simulink model "IEEE_1547_UI_TEST"  (R2018b)
settings: Solver=ode4  StartTime=0.0  StopTime=inf  FixedStep=Ts  RelTol=1e-3  EnableMultiTasking=on
PostLoadFcn:
  | Ts=40e-6; ARTEMIS_DISABLE_RTLAB_COMPATIBILTY_CHECK=1;
InitFcn:
  | Ts=40e-6; ARTEMIS_DISABLE_RTLAB_COMPATIBILTY_CHECK=1;
undefined symbols (not defined in the file or in its folder): another_event_name, I, Left, my_event_name, Right, type, V
libraries: simulink x72, powerlib_meascontrol x70, powerlib x66, artemis x4, rtlab x3, rtio_opalrt_ml605ex1 x3
(part 3 of 3)

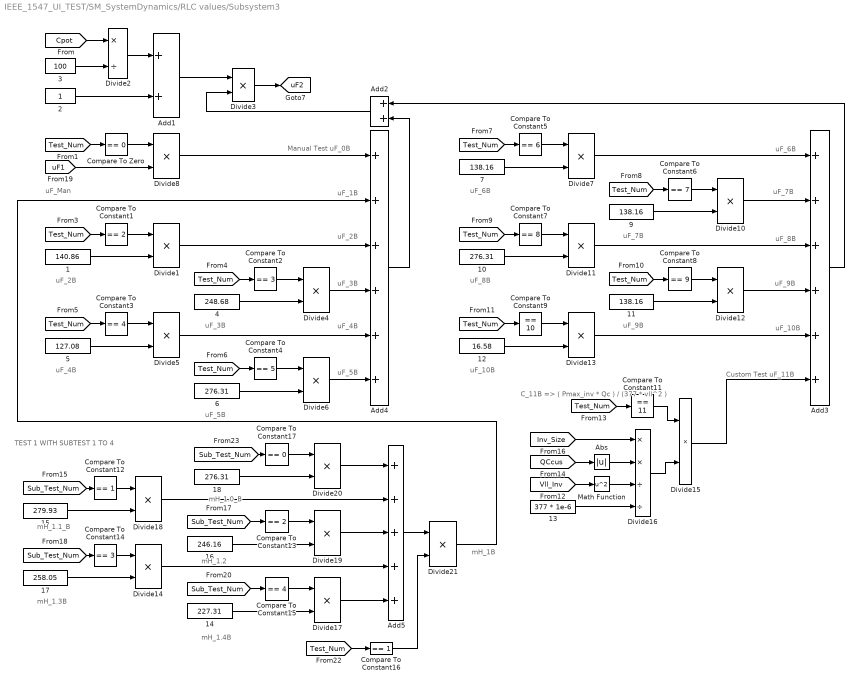
== system IEEE_1547_UI_TEST/SM_SystemDynamics/RLC values/Subsystem3 ==
  note: uF_8B
  note: uF_7B
  note: Manual Test uF_0B
  note: Custom Test uF_11B
  note: uF_2B
  note: uF_7B
  note: mH_1B
  note: uF_8B
  note: uF_5B
  note: C_11B => ( Pmax_inv * Qc ) / (377 * vll^2 )
  note: uF_6B
  note: uF_Man
  note: mH_1.0_B
  note: uF_4B
  note: uF_10B
  note: mH_1.3B
  note: uF_4B
  note: uF_9B
  note: mH_1.2
  note: mH_1.4B
  note: uF_2B
  note: TEST 1 WITH SUBTEST 1 TO 4
  note: uF_9B
  note: uF_5B
  note: uF_10B
  note: uF_6B
  note: uF_3B
  note: uF_3B
  note: mH_1.1_B
  note: uF_1B
  1 : Constant  Value=140.86
  10 : Constant  Value=276.31
  11 : Constant  Value=138.16
  12 : Constant  Value=16.58
  13 : Constant  Value=377 * 1e-6
  14 : Constant  Value=227.31
  15 : Constant  Value=279.93
  16 : Constant  Value=246.16
  17 : Constant  Value=258.05
  18 : Constant  Value=276.31
  2 : Constant
  3 : Constant  Value=100
  4 : Constant  Value=248.68
  5 : Constant  Value=127.08
  6 : Constant  Value=276.31
  7 : Constant  Value=138.16
  9 : Constant  Value=138.16
  Abs : Abs
  Add1 : Sum
  Add2 : Sum
  Add3 : Sum  Inputs=++++++
  Add4 : Sum  Inputs=++++++
  Add5 : Sum  Inputs=+++++
  Compare To Constant1 : simulink/Logic and Bit Operations/Compare To Constant  relop===  const=2  OutDataTypeStr=boolean
  Compare To Constant11 : simulink/Logic and Bit Operations/Compare To Constant  relop===  const=11  OutDataTypeStr=boolean
  Compare To Constant12 : simulink/Logic and Bit Operations/Compare To Constant  relop===  const=1  OutDataTypeStr=boolean
  Compare To Constant13 : simulink/Logic and Bit Operations/Compare To Constant  relop===  const=2  OutDataTypeStr=boolean
  Compare To Constant14 : simulink/Logic and Bit Operations/Compare To Constant  relop===  const=3  OutDataTypeStr=boolean
  Compare To Constant15 : simulink/Logic and Bit Operations/Compare To Constant  relop===  const=4  OutDataTypeStr=boolean
  Compare To Constant16 : simulink/Logic and Bit Operations/Compare To Constant  relop===  const=1  OutDataTypeStr=boolean
  Compare To Constant17 : simulink/Logic and Bit Operations/Compare To Constant  relop===  const=0  OutDataTypeStr=boolean
  Compare To Constant2 : simulink/Logic and Bit Operations/Compare To Constant  relop===  const=3  OutDataTypeStr=boolean
  Compare To Constant3 : simulink/Logic and Bit Operations/Compare To Constant  relop===  const=4  OutDataTypeStr=boolean
  Compare To Constant4 : simulink/Logic and Bit Operations/Compare To Constant  relop===  const=5  OutDataTypeStr=boolean
  Compare To Constant5 : simulink/Logic and Bit Operations/Compare To Constant  relop===  const=6  OutDataTypeStr=boolean
  Compare To Constant6 : simulink/Logic and Bit Operations/Compare To Constant  relop===  const=7  OutDataTypeStr=boolean
  Compare To Constant7 : simulink/Logic and Bit Operations/Compare To Constant  relop===  const=8  OutDataTypeStr=boolean
  Compare To Constant8 : simulink/Logic and Bit Operations/Compare To Constant  relop===  const=9  OutDataTypeStr=boolean
  Compare To Constant9 : simulink/Logic and Bit Operations/Compare To Constant  relop===  const=10  OutDataTypeStr=boolean
  Compare To Zero : simulink/Logic and Bit Operations/Compare To Zero  relop===  OutDataTypeStr=boolean
  Divide{1,3..8,10..15,17..21} (18 alike) : Product  Inputs=**
  Divide16 : Product  Inputs=**//
  Divide2 : Product  Inputs=*/
  Math Function : Math  Operator=square  SaturateOnIntegerOverflow=on
  tag scope: uF2=global
  wires:
  [Test_Num] -> Compare To Constant9/1
  Compare To Constant5/1 -> Divide7/1
  Divide3/1 -> [uF2]
  [Sub_Test_Num] -> Compare To Constant15/1
  Divide21/1 -> Add4/2
  Divide17/1 -> Add5/5
  [Test_Num] -> Compare To Constant7/1
  Divide19/1 -> Add5/3
  11/1 -> Divide12/2
  Compare To Constant17/1 -> Divide20/1
  14/1 -> Divide17/2
  Compare To Constant16/1 -> Divide21/2
  Add5/1 -> Divide21/1
  5/1 -> Divide5/2
  Divide12/1 -> Add3/4
  Divide8/1 -> Add4/1
  Compare To Constant14/1 -> Divide14/1
  Compare To Constant6/1 -> Divide10/1
  16/1 -> Divide19/2
  15/1 -> Divide18/2
  Compare To Constant12/1 -> Divide18/1
  13/1 -> Divide16/4
  [Sub_Test_Num] -> Compare To Constant14/1
  Divide20/1 -> Add5/1
  Abs/1 -> Divide16/2
  Compare To Constant15/1 -> Divide17/1
  Divide6/1 -> Add4/6
  10/1 -> Divide11/2
  6/1 -> Divide6/2
  [Test_Num] -> Compare To Constant8/1
  [Inv_Size] -> Divide16/1
  [Sub_Test_Num] -> Compare To Constant13/1
  Add4/1 -> Add2/2
  Compare To Constant1/1 -> Divide1/1
  Add2/1 -> Divide3/2
  Compare To Constant11/1 -> Divide15/1
  Divide16/1 -> Divide15/2
  Compare To Constant8/1 -> Divide12/1
  3/1 -> Divide2/2
  Compare To Constant13/1 -> Divide19/1
  12/1 -> Divide13/2
  Math Function/1 -> Divide16/3
  Divide10/1 -> Add3/2
  Divide2/1 -> Add1/1
  Divide4/1 -> Add4/4
  Divide14/1 -> Add5/4
  Divide13/1 -> Add3/5
  [Test_Num] -> Compare To Constant11/1
  Divide5/1 -> Add4/5
  Compare To Constant7/1 -> Divide11/1
  [QCcus] -> Abs/1
  Compare To Constant2/1 -> Divide4/1
  Compare To Constant4/1 -> Divide6/1
  [Test_Num] -> Compare To Constant6/1
  Divide15/1 -> Add3/6
  Compare To Zero/1 -> Divide8/1
  Add3/1 -> Add2/1
  Divide11/1 -> Add3/3
  Compare To Constant9/1 -> Divide13/1
  7/1 -> Divide7/2
  9/1 -> Divide10/2
  [Test_Num] -> Compare To Constant5/1
  17/1 -> Divide14/2
  [Test_Num] -> Compare To Constant2/1
  [Test_Num] -> Compare To Constant3/1
  18/1 -> Divide20/2
  [Sub_Test_Num] -> Compare To Constant17/1
  Divide1/1 -> Add4/3
  [Test_Num] -> Compare To Constant16/1
  [Test_Num] -> Compare To Constant1/1
  2/1 -> Add1/2
  1/1 -> Divide1/2
  Compare To Constant3/1 -> Divide5/1
  Divide18/1 -> Add5/2
  [Test_Num] -> Compare To Zero/1
  [Vll_Inv] -> Math Function/1
  [Test_Num] -> Compare To Constant4/1
  Add1/1 -> Divide3/1
  Divide7/1 -> Add3/1
  [Sub_Test_Num] -> Compare To Constant12/1
  4/1 -> Divide4/2
  [Cpot] -> Divide2/1
  [uF1] -> Divide8/2

== system IEEE_1547_UI_TEST/SM_SystemDynamics/Subsystem8/AVG( RMS )1 ==
  In1 : Inport
  Mean : powerlib_meascontrol/Measurements/Mean  Freq=60  Vinit=0  Ts=Ts
      settings: SourceProductName=Simscape Electrical
  RMS : powerlib_meascontrol/Measurements/RMS  TrueRMS=on  Freq=60  RMSInit=120  Ts=Ts
      settings: SourceProductName=Simscape Electrical
  Out1 : Outport
  wires:
  Mean/1 -> Out1/1
  RMS/1 -> Mean/1
  In1/1 -> RMS/1

== system IEEE_1547_UI_TEST/SM_SystemDynamics/Subsystem8/AVG( RMS )4 ==
  In1 : Inport
  Mean : powerlib_meascontrol/Measurements/Mean  Freq=60  Vinit=0  Ts=Ts
      settings: SourceProductName=Simscape Electrical
  RMS : powerlib_meascontrol/Measurements/RMS  TrueRMS=on  Freq=60  RMSInit=120  Ts=Ts
      settings: SourceProductName=Simscape Electrical
  Out1 : Outport
  wires:
  Mean/1 -> Out1/1
  RMS/1 -> Mean/1
  In1/1 -> RMS/1

== system IEEE_1547_UI_TEST/SM_SystemDynamics/Subsystem8/Phase Angle Meter1 ==
  Vabc : Inport
  Iabc : Inport  Port=2
  Constant : Constant  Value=-1
  Cos : Trigonometry  Operator=cos
  Gain : Gain  Gain=pi/180
  PLL (3ph) : powerlib_meascontrol/PLL/PLL (3ph)  Fmin=30  Par_Init=[0, 60]  ParK=[180, 3200, 1]  TcD=1e-4  MaxRateChangeFreq=12  FilterCutOffFreq=25  Ts=Ts  AGC=on
  Positive-Sequence (PLL-Driven) : powerlib_meascontrol/Measurements/Positive-Sequence (PLL-Driven)  Finit=60  Fmin=45  InInit=[1, 0]  Ts=Ts
      settings: SourceProductName=Simscape Power Systems  SourceProductBaseCode=PS
  Product : Product  Inputs=3
  Sign : Signum
  Θ : Outport
  pf : Outport  Port=2
  wires:
  PLL (3ph)/1 -> Positive-Sequence (PLL-Driven)/1
  PLL (3ph)/2 -> Positive-Sequence (PLL-Driven)/2
  Iabc/1 -> Positive-Sequence (PLL-Driven)/3
  Vabc/1 -> PLL (3ph)/1
  Positive-Sequence (PLL-Driven)/2 -> Gain/1, Sign/1, Θ/1
  Product/1 -> pf/1
  Gain/1 -> Cos/1
  Cos/1 -> Product/3
  Sign/1 -> Product/1
  Constant/1 -> Product/2

== system IEEE_1547_UI_TEST/SM_SystemDynamics/Subsystem8/Power, 3Ph ( Fundamental Frecuency )1 ==
  Vabc : Inport
  Iabc : Inport  Port=2
  Inv Size : Inport  Port=3
  Divide : Product  Inputs=*/
  Divide1 : Product  Inputs=*/
  Mean1 : powerlib_meascontrol/Measurements/Mean  Freq=30  Vinit=0  Ts=Ts
      settings: SourceProductName=Simscape Electrical
  Mean2 : powerlib_meascontrol/Measurements/Mean  Freq=30  Vinit=0  Ts=Ts
      settings: SourceProductName=Simscape Electrical
  PLL (3ph) : powerlib_meascontrol/PLL/PLL (3ph)  Fmin=45  Par_Init=[0, 60]  ParK=[180, 3200, 1]  TcD=1e-4  MaxRateChangeFreq=12  FilterCutOffFreq=25  Ts=Ts  AGC=on
      settings: SourceProductName=Simscape Electrical
  Power ( Fundamental Frecuency ) : powerlib_meascontrol/Measurements/Power (PLL-Driven, Positive-Sequence)  Finit=60  Fmin=45  Vinit=[1, 0]  Iinit=[1, 0]  Ts=Ts
      settings: SourceProductName=Simscape Electrical  SourceProductBaseCode=PS
  P_Load_Watts : Outport
  Q_Load_Vars : Outport  Port=2
  P_Load_pu : Outport  Port=3
  Q_Load_pu : Outport  Port=4
  Freq_PCC : Outport  Port=5
  wires:
  Mean2/1 -> P_Load_Watts/1, Divide/1
  Inv Size/1 -> Divide/2, Divide1/2
  Power ( Fundamental Frecuency )/1 -> Mean2/1
  Mean1/1 -> Divide1/1, Q_Load_Vars/1
  Power ( Fundamental Frecuency )/2 -> Mean1/1
  Divide/1 -> P_Load_pu/1
  Divide1/1 -> Q_Load_pu/1
  PLL (3ph)/1 -> Freq_PCC/1, Power ( Fundamental Frecuency )/1
  PLL (3ph)/2 -> Power ( Fundamental Frecuency )/2
  Vabc/1 -> Power ( Fundamental Frecuency )/3, PLL (3ph)/1
  Iabc/1 -> Power ( Fundamental Frecuency )/4

== system IEEE_1547_UI_TEST/SM_SystemDynamics/UTILITY1/AVG( RMS )4 ==
  In1 : Inport
  Mean : powerlib_meascontrol/Measurements/Mean  Freq=60  Vinit=0  Ts=Ts
      settings: SourceProductName=Simscape Electrical
  RMS : powerlib_meascontrol/Measurements/RMS  TrueRMS=on  Freq=60  RMSInit=120  Ts=Ts
      settings: SourceProductName=Simscape Electrical
  Out1 : Outport
  wires:
  Mean/1 -> Out1/1
  RMS/1 -> Mean/1
  In1/1 -> RMS/1

== system IEEE_1547_UI_TEST/SM_SystemDynamics/UTILITY1/AVG( RMS )5 ==
  In1 : Inport
  Mean : powerlib_meascontrol/Measurements/Mean  Freq=60  Vinit=0  Ts=Ts
      settings: SourceProductName=Simscape Electrical
  RMS : powerlib_meascontrol/Measurements/RMS  TrueRMS=on  Freq=60  RMSInit=120  Ts=Ts
      settings: SourceProductName=Simscape Electrical
  Out1 : Outport
  wires:
  Mean/1 -> Out1/1
  RMS/1 -> Mean/1
  In1/1 -> RMS/1

== system IEEE_1547_UI_TEST/SM_SystemDynamics/UTILITY1/Power, 3Ph ( Fundamental Frecuency )2 ==
  Vabc : Inport
  Iabc : Inport  Port=2
  Inv Size : Inport  Port=3
  Divide : Product  Inputs=*/
  Divide1 : Product  Inputs=*/
  Gain : Gain
  Gain1 : Gain
  Mean{1..4} (4 alike) : powerlib_meascontrol/Measurements/Mean  Freq=30  Vinit=0  Ts=Ts
      settings: SourceProductName=Simscape Electrical
  PLL (3ph) : powerlib_meascontrol/PLL/PLL (3ph)  Fmin=45  Par_Init=[0, 60]  ParK=[180, 3200, 1]  TcD=1e-4  MaxRateChangeFreq=12  FilterCutOffFreq=25  Ts=Ts  AGC=on
      settings: SourceProductName=Simscape Electrical
  Power ( Fundamental Frecuency ) : powerlib_meascontrol/Measurements/Power (PLL-Driven, Positive-Sequence)  Finit=60  Fmin=45  Vinit=[1, 0]  Iinit=[1, 0]  Ts=Ts
      settings: SourceProductName=Simscape Electrical  SourceProductBaseCode=PS
  Pt_uti_Watts : Outport
  Quti_Vars : Outport  Port=2
  Puti_pu : Outport  Port=3
  Quti_pu : Outport  Port=4
  Freq_EPS : Outport  Port=5
  wires:
  Mean2/1 -> Divide/1
  Gain/1 -> Divide/2
  Power ( Fundamental Frecuency )/1 -> Mean3/1, Mean2/1
  Mean1/1 -> Divide1/1
  Gain1/1 -> Divide1/2
  Power ( Fundamental Frecuency )/2 -> Mean4/1, Mean1/1
  Divide/1 -> Puti_pu/1
  Divide1/1 -> Quti_pu/1
  Inv Size/1 -> Gain/1, Gain1/1
  PLL (3ph)/1 -> Freq_EPS/1, Power ( Fundamental Frecuency )/1
  PLL (3ph)/2 -> Power ( Fundamental Frecuency )/2
  Iabc/1 -> Power ( Fundamental Frecuency )/4
  Mean3/1 -> Pt_uti_Watts/1
  Mean4/1 -> Quti_Vars/1
  Vabc/1 -> Power ( Fundamental Frecuency )/3, PLL (3ph)/1

== system IEEE_1547_UI_TEST/SM_SystemDynamics/ 3Phase Y Load with N/   C Bank/AVG( RMS )1 ==
  In1 : Inport
  Mean : powerlib_meascontrol/Measurements/Mean  Freq=60  Vinit=0  Ts=Ts
      settings: SourceProductName=Simscape Electrical
  RMS : powerlib_meascontrol/Measurements/RMS  TrueRMS=on  Freq=60  RMSInit=120  Ts=Ts
      settings: SourceProductName=Simscape Electrical
  Out1 : Outport
  wires:
  Mean/1 -> Out1/1
  RMS/1 -> Mean/1
  In1/1 -> RMS/1

== system IEEE_1547_UI_TEST/SM_SystemDynamics/ 3Phase Y Load with N/   C Bank/C1 ==
  note: C
  note: Ic
  note: ic(t)
  note: Vc(t)
  note: dVc(t)
      | -------
      |    dt
  note: Capacitor Equations
      |
      | Ic = C dVc/dt
      |
      | dVc/dt = 1/C * Ic
  uC : Inport
  1 micro ohm : powerlib/Elements/Series RLC Branch  LConnTagsString=__new0  RConnTagsString=__new0  BranchType=R  Resistance=1e-6  Inductance=1e-3  SetiL0=off  InitialCurrent=0  Capacitance=1e-6  Setx0=off  InitialVoltage=0  Measurements=None
      settings: SourceProductName=Simscape Electrical
  1/L3 : Product  Inputs=*/  SaturateOnIntegerOverflow=on  OutDataTypeStr=Inherit: Same as first input
  Constant2 : Constant  Value=1e-6
  Controlled Voltage Source2 : powerlib/Electrical Sources/Controlled Voltage Source  Initialize=on  Source_Type=AC  Amplitude=277  Phase=0  Frequency=0  Measurements=None
      settings: SourceProductName=Simscape Electrical
  Divide2 : Product  Inputs=**
  Integrator2 : Integrator
  Vc : powerlib/Measurements/Voltage Measurement  PhasorSimulation=off  OutputType=Magnitude  PSBequivalent=0
      settings: SourceProductName=Simscape Electrical
  it(t)2 : powerlib/Measurements/Current Measurement  PhasorSimulation=off  OutputType=Complex  PSBequivalent=0
      settings: SourceProductName=Simscape Electrical
  ohms Limiter3 : Saturate  UpperLimit=inf  LowerLimit=1e-9
  V+ : PMIOPort  Side=Right
  V- : PMIOPort  Port=2  Side=Right
  V_C : Outport
  I_C : Outport  Port=2
  wires:
  Integrator2/1 -> Controlled Voltage Source2/1
  Vc/1 -> V_C/1
  Divide2/1 -> 1/L3/2
  uC/1 -> ohms Limiter3/1
  ohms Limiter3/1 -> Divide2/2
  Constant2/1 -> Divide2/1
  1/L3/1 -> Integrator2/1
  it(t)2/1 -> I_C/1, 1/L3/1
  connections:
  Vc/LConn2 -- Controlled Voltage Source2/LConn1 -- V-/RConn1
  Vc/LConn1 -- it(t)2/LConn1 -- V+/RConn1
  1 micro ohm/LConn1 -- Controlled Voltage Source2/RConn1
  it(t)2/RConn1 -- 1 micro ohm/RConn1

== system IEEE_1547_UI_TEST/SM_SystemDynamics/ 3Phase Y Load with N/   C Bank/C2 ==
  note: C
  note: Ic
  note: ic(t)
  note: Vc(t)
  note: dVc(t)
      | -------
      |    dt
  note: Capacitor Equations
      |
      | Ic = C dVc/dt
      |
      | dVc/dt = 1/C * Ic
  uC : Inport
  1 micro ohm : powerlib/Elements/Series RLC Branch  LConnTagsString=__new0  RConnTagsString=__new0  BranchType=R  Resistance=1e-6  Inductance=1e-3  SetiL0=off  InitialCurrent=0  Capacitance=1e-6  Setx0=off  InitialVoltage=0  Measurements=None
      settings: SourceProductName=Simscape Electrical
  1/L3 : Product  Inputs=*/  SaturateOnIntegerOverflow=on  OutDataTypeStr=Inherit: Same as first input
  Constant2 : Constant  Value=1e-6
  Controlled Voltage Source2 : powerlib/Electrical Sources/Controlled Voltage Source  Initialize=on  Source_Type=AC  Amplitude=277  Phase=0  Frequency=0  Measurements=None
      settings: SourceProductName=Simscape Electrical
  Divide2 : Product  Inputs=**
  Integrator2 : Integrator
  Vc : powerlib/Measurements/Voltage Measurement  PhasorSimulation=off  OutputType=Magnitude  PSBequivalent=0
      settings: SourceProductName=Simscape Electrical
  it(t)2 : powerlib/Measurements/Current Measurement  PhasorSimulation=off  OutputType=Complex  PSBequivalent=0
      settings: SourceProductName=Simscape Electrical
  ohms Limiter3 : Saturate  UpperLimit=inf  LowerLimit=1e-9
  V+ : PMIOPort  Side=Right
  V- : PMIOPort  Port=2  Side=Right
  V_C : Outport
  I_C : Outport  Port=2
  wires:
  Integrator2/1 -> Controlled Voltage Source2/1
  Vc/1 -> V_C/1
  Divide2/1 -> 1/L3/2
  uC/1 -> ohms Limiter3/1
  ohms Limiter3/1 -> Divide2/2
  Constant2/1 -> Divide2/1
  1/L3/1 -> Integrator2/1
  it(t)2/1 -> I_C/1, 1/L3/1
  connections:
  Vc/LConn2 -- Controlled Voltage Source2/LConn1 -- V-/RConn1
  Vc/LConn1 -- it(t)2/LConn1 -- V+/RConn1
  1 micro ohm/LConn1 -- Controlled Voltage Source2/RConn1
  it(t)2/RConn1 -- 1 micro ohm/RConn1

== system IEEE_1547_UI_TEST/SM_SystemDynamics/ 3Phase Y Load with N/   C Bank/C3 ==
  note: C
  note: Ic
  note: ic(t)
  note: Vc(t)
  note: dVc(t)
      | -------
      |    dt
  note: Capacitor Equations
      |
      | Ic = C dVc/dt
      |
      | dVc/dt = 1/C * Ic
  uC : Inport
  1 micro ohm : powerlib/Elements/Series RLC Branch  LConnTagsString=__new0  RConnTagsString=__new0  BranchType=R  Resistance=1e-6  Inductance=1e-3  SetiL0=off  InitialCurrent=0  Capacitance=1e-6  Setx0=off  InitialVoltage=0  Measurements=None
      settings: SourceProductName=Simscape Electrical
  1/L3 : Product  Inputs=*/  SaturateOnIntegerOverflow=on  OutDataTypeStr=Inherit: Same as first input
  Constant2 : Constant  Value=1e-6
  Controlled Voltage Source2 : powerlib/Electrical Sources/Controlled Voltage Source  Initialize=on  Source_Type=AC  Amplitude=277  Phase=0  Frequency=0  Measurements=None
      settings: SourceProductName=Simscape Electrical
  Divide2 : Product  Inputs=**
  Integrator2 : Integrator
  Vc : powerlib/Measurements/Voltage Measurement  PhasorSimulation=off  OutputType=Magnitude  PSBequivalent=0
      settings: SourceProductName=Simscape Electrical
  it(t)2 : powerlib/Measurements/Current Measurement  PhasorSimulation=off  OutputType=Complex  PSBequivalent=0
      settings: SourceProductName=Simscape Electrical
  ohms Limiter3 : Saturate  UpperLimit=inf  LowerLimit=1e-9
  V+ : PMIOPort  Side=Right
  V- : PMIOPort  Port=2  Side=Right
  V_C : Outport
  I_C : Outport  Port=2
  wires:
  Integrator2/1 -> Controlled Voltage Source2/1
  Vc/1 -> V_C/1
  Divide2/1 -> 1/L3/2
  uC/1 -> ohms Limiter3/1
  ohms Limiter3/1 -> Divide2/2
  Constant2/1 -> Divide2/1
  1/L3/1 -> Integrator2/1
  it(t)2/1 -> I_C/1, 1/L3/1
  connections:
  Vc/LConn2 -- Controlled Voltage Source2/LConn1 -- V-/RConn1
  Vc/LConn1 -- it(t)2/LConn1 -- V+/RConn1
  1 micro ohm/LConn1 -- Controlled Voltage Source2/RConn1
  it(t)2/RConn1 -- 1 micro ohm/RConn1

== system IEEE_1547_UI_TEST/SM_SystemDynamics/ 3Phase Y Load with N/   C Bank/Power per Element ==
  Vabc : Inport
  Iabc : Inport  Port=2
  Demux : Demux  Outputs=3
  Demux1 : Demux  Outputs=3
  Demux2 : Demux  Outputs=6
  Divide : Product  Inputs=*/
  Gain : Gain  Gain=-1/3
  Mux : Mux  Inputs=6
  Power1 : powerlib_meascontrol/Measurements/Power  Freq=60  Vinit=[1, 0]  Iinit=[1, 0]  Ts=Ts
      settings: SourceProductName=Simscape Power Systems
  Power2 : powerlib_meascontrol/Measurements/Power  Freq=60  Vinit=[1, 0]  Iinit=[1, 0]  Ts=Ts
      settings: SourceProductName=Simscape Power Systems
  Power3 : powerlib_meascontrol/Measurements/Power  Freq=60  Vinit=[1, 0]  Iinit=[1, 0]  Ts=Ts
      settings: SourceProductName=Simscape Power Systems
  tag scope: C1_P=global, C1_Q=global, C2_P=global, C2_Q=global, C3_P=global, C3_Q=global
  wires:
  Demux1/2 -> Power2/2
  Demux/1 -> Power1/1
  Demux1/3 -> Power3/2
  Demux/2 -> Power2/1
  Demux/3 -> Power3/1
  Demux1/1 -> Power1/2
  Iabc/1 -> Demux1/1
  Vabc/1 -> Demux/1
  Demux2/6 -> [C3_Q]
  Power1/1 -> Mux/1
  Power1/2 -> Mux/2
  [Inv_Size] -> Gain/1
  Demux2/3 -> [C2_P]
  Demux2/2 -> [C1_Q]
  Demux2/5 -> [C3_P]
  Demux2/4 -> [C2_Q]
  Divide/1 -> Demux2/1
  Mux/1 -> Divide/1
  Demux2/1 -> [C1_P]
  Power2/1 -> Mux/3
  Power3/2 -> Mux/6
  Power2/2 -> Mux/4
  Power3/1 -> Mux/5
  Gain/1 -> Divide/2

== system IEEE_1547_UI_TEST/SM_SystemDynamics/ 3Phase Y Load with N/   C Bank/Power, 3Ph (  Fund. Frecu. ) ==
  note: Per Unit Converter
  Vabc : Inport
  Iabc : Inport  Port=2
  Divide : Product  Inputs=*/
  Divide1 : Product  Inputs=*/
  Gain : Gain  Gain=-1
  Gain1 : Gain  Gain=-1
  Mean : powerlib_meascontrol/Measurements/Mean  Freq=30  Vinit=0  Ts=Ts
      settings: SourceProductName=Simscape Electrical
  Mean1 : powerlib_meascontrol/Measurements/Mean  Freq=30  Vinit=0  Ts=Ts
      settings: SourceProductName=Simscape Electrical
  PLL (3ph) : powerlib_meascontrol/PLL/PLL (3ph)  Fmin=60  Par_Init=[0, 60]  ParK=[180, 3200, 1]  TcD=1e-4  MaxRateChangeFreq=12  FilterCutOffFreq=25  Ts=Ts  AGC=on
      settings: SourceProductName=Simscape Electrical
  Power ( Fundamental Frecuency ) : powerlib_meascontrol/Measurements/Power (PLL-Driven, Positive-Sequence)  Finit=60  Fmin=45  Vinit=[1, 0]  Iinit=[1, 0]  Ts=Ts
      settings: SourceProductName=Simscape Electrical  SourceProductBaseCode=PS
  P : Outport
  Q : Outport  Port=2
  wires:
  Mean/1 -> Divide/1
  [Inv_Size] -> Gain/1
  Gain/1 -> Divide/2
  Power ( Fundamental Frecuency )/2 -> Mean/1
  Power ( Fundamental Frecuency )/1 -> Mean1/1
  Divide/1 -> Q/1
  Mean1/1 -> Divide1/1
  [Inv_Size] -> Gain1/1
  Gain1/1 -> Divide1/2
  Divide1/1 -> P/1
  PLL (3ph)/1 -> Power ( Fundamental Frecuency )/1
  PLL (3ph)/2 -> Power ( Fundamental Frecuency )/2
  Vabc/1 -> Power ( Fundamental Frecuency )/3, PLL (3ph)/1
  Iabc/1 -> Power ( Fundamental Frecuency )/4

== system IEEE_1547_UI_TEST/SM_SystemDynamics/ 3Phase Y Load with N/   R Bank1/3Ph ( P.U. ) Power, Fund. Frec. ==
  Vabc : Inport
  Iabc : Inport  Port=2
  Divide : Product  Inputs=*/
  Gain : Gain  Gain=-1
  Mean : powerlib_meascontrol/Measurements/Mean  Freq=30  Vinit=0  Ts=Ts
      settings: SourceProductName=Simscape Electrical
  Mean1 : powerlib_meascontrol/Measurements/Mean  Freq=30  Vinit=0  Ts=Ts
      settings: SourceProductName=Simscape Electrical
  PLL (3ph) : powerlib_meascontrol/PLL/PLL (3ph)  Fmin=60  Par_Init=[0, 60]  ParK=[180, 3200, 1]  TcD=1e-4  MaxRateChangeFreq=12  FilterCutOffFreq=25  Ts=Ts  AGC=on
      settings: SourceProductName=Simscape Electrical
  Power ( Fundamental Frecuency ) : powerlib_meascontrol/Measurements/Power (PLL-Driven, Positive-Sequence)  Finit=60  Fmin=45  Vinit=[1, 0]  Iinit=[1, 0]  Ts=Ts
      settings: SourceProductName=Simscape Electrical  SourceProductBaseCode=PS
  P : Outport
  Q : Outport  Port=2
  wires:
  PLL (3ph)/2 -> Power ( Fundamental Frecuency )/2
  PLL (3ph)/1 -> Power ( Fundamental Frecuency )/1
  Power ( Fundamental Frecuency )/2 -> Mean1/1
  Power ( Fundamental Frecuency )/1 -> Mean/1
  Iabc/1 -> Power ( Fundamental Frecuency )/4
  Vabc/1 -> PLL (3ph)/1, Power ( Fundamental Frecuency )/3
  Mean/1 -> Divide/1
  Mean1/1 -> Q/1
  [Inv_Size] -> Gain/1
  Divide/1 -> P/1
  Gain/1 -> Divide/2

== system IEEE_1547_UI_TEST/SM_SystemDynamics/ 3Phase Y Load with N/   R Bank1/AVG( RMS )4 ==
  In1 : Inport
  Mean : powerlib_meascontrol/Measurements/Mean  Freq=60  Vinit=0  Ts=Ts
      settings: SourceProductName=Simscape Electrical
  RMS : powerlib_meascontrol/Measurements/RMS  TrueRMS=on  Freq=60  RMSInit=120  Ts=Ts
      settings: SourceProductName=Simscape Electrical
  Out1 : Outport
  wires:
  Mean/1 -> Out1/1
  RMS/1 -> Mean/1
  In1/1 -> RMS/1

== system IEEE_1547_UI_TEST/SM_SystemDynamics/ 3Phase Y Load with N/   R Bank1/Power per Element ==
  Vabc : Inport
  Iabc : Inport  Port=2
  Demux : Demux  Outputs=3
  Demux1 : Demux  Outputs=3
  Demux2 : Demux  Outputs=6
  Divide : Product  Inputs=*/
  Gain : Gain  Gain=-1/3
  Mux : Mux  Inputs=6
  Power1 : powerlib_meascontrol/Measurements/Power  Freq=60  Vinit=[1, 0]  Iinit=[1, 0]  Ts=Ts
      settings: SourceProductName=Simscape Power Systems
  Power2 : powerlib_meascontrol/Measurements/Power  Freq=60  Vinit=[1, 0]  Iinit=[1, 0]  Ts=Ts
      settings: SourceProductName=Simscape Power Systems
  Power3 : powerlib_meascontrol/Measurements/Power  Freq=60  Vinit=[1, 0]  Iinit=[1, 0]  Ts=Ts
      settings: SourceProductName=Simscape Power Systems
  tag scope: R1_P=global, R1_Q=global, R2_P=global, R2_Q=global, R3_P=global, R3_Q=global
  wires:
  Power1/1 -> Mux/1
  Demux1/2 -> Power2/2
  Demux/1 -> Power1/1
  Demux1/3 -> Power3/2
  Demux/2 -> Power2/1
  Demux/3 -> Power3/1
  Power2/1 -> Mux/3
  Power2/2 -> Mux/4
  Power3/1 -> Mux/5
  Demux1/1 -> Power1/2
  Power3/2 -> Mux/6
  Power1/2 -> Mux/2
  Iabc/1 -> Demux1/1
  Vabc/1 -> Demux/1
  Gain/1 -> Divide/2
  [Inv_Size] -> Gain/1
  Mux/1 -> Divide/1
  Divide/1 -> Demux2/1
  Demux2/1 -> [R1_P]
  Demux2/2 -> [R1_Q]
  Demux2/3 -> [R2_P]
  Demux2/4 -> [R2_Q]
  Demux2/5 -> [R3_P]
  Demux2/6 -> [R3_Q]

== system IEEE_1547_UI_TEST/SM_SystemDynamics/ 3Phase Y Load with N/   R Bank1/R1 ==
  note: I R = V / R
  note: 10
      | Mohms
  ohms : Inport
  Controlled Current Source : powerlib/Electrical Sources/Controlled Current Source  Initialize=on  Source_Type=AC  Amplitude=0  Phase=0  Frequency=0  Measurements=None
      settings: SourceProductName=Simscape Electrical
  Divide : Product  Inputs=/*
  Memory : Memory  InitialCondition=10
  Series RLC Branch1 : powerlib/Elements/Series RLC Branch  LConnTagsString=__new0  RConnTagsString=__new0  BranchType=R  Resistance=10e6  Inductance=1e-3  SetiL0=off  InitialCurrent=0  Capacitance=1e-6  Setx0=off  InitialVoltage=0  Measurements=None
      settings: SourceProductName=Simscape Electrical
  Voltage Measurement : powerlib/Measurements/Voltage Measurement  PhasorSimulation=off  OutputType=Complex  PSBequivalent=0
      settings: SourceProductName=Simscape Electrical
  ic(t) : powerlib/Measurements/Current Measurement  PhasorSimulation=off  OutputType=Complex  PSBequivalent=0
      settings: SourceProductName=Simscape Electrical
  ohms Limiter : Saturate  UpperLimit=100e6  LowerLimit=0.001
  Lin : PMIOPort  Side=Right
  Lout : PMIOPort  Port=2  Side=Right
  V : Outport
  I : Outport  Port=2
  wires:
  Memory/1 -> V/1, Divide/2
  ic(t)/1 -> I/1
  Divide/1 -> Controlled Current Source/1
  Voltage Measurement/1 -> Memory/1
  ohms Limiter/1 -> Divide/1
  ohms/1 -> ohms Limiter/1
  connections:
  Lin/RConn1 -- Controlled Current Source/LConn1 -- Voltage Measurement/LConn1 -- Series RLC Branch1/LConn1
  Lout/RConn1 -- Voltage Measurement/LConn2 -- ic(t)/RConn1 -- Series RLC Branch1/RConn1
  Controlled Current Source/RConn1 -- ic(t)/LConn1

== system IEEE_1547_UI_TEST/SM_SystemDynamics/ 3Phase Y Load with N/   R Bank1/R2 ==
  note: I R = V / R
  note: 10
      | Mohms
  ohms : Inport
  Controlled Current Source : powerlib/Electrical Sources/Controlled Current Source  Initialize=on  Source_Type=AC  Amplitude=0  Phase=0  Frequency=0  Measurements=None
      settings: SourceProductName=Simscape Electrical
  Divide : Product  Inputs=/*
  Memory : Memory  InitialCondition=10
  Series RLC Branch1 : powerlib/Elements/Series RLC Branch  LConnTagsString=__new0  RConnTagsString=__new0  BranchType=R  Resistance=10e6  Inductance=1e-3  SetiL0=off  InitialCurrent=0  Capacitance=1e-6  Setx0=off  InitialVoltage=0  Measurements=None
      settings: SourceProductName=Simscape Electrical
  Voltage Measurement : powerlib/Measurements/Voltage Measurement  PhasorSimulation=off  OutputType=Complex  PSBequivalent=0
      settings: SourceProductName=Simscape Electrical
  ic(t) : powerlib/Measurements/Current Measurement  PhasorSimulation=off  OutputType=Complex  PSBequivalent=0
      settings: SourceProductName=Simscape Electrical
  ohms Limiter : Saturate  UpperLimit=100e6  LowerLimit=0.001
  Lin : PMIOPort  Side=Right
  Lout : PMIOPort  Port=2  Side=Right
  V : Outport
  I : Outport  Port=2
  wires:
  Memory/1 -> V/1, Divide/2
  ic(t)/1 -> I/1
  Divide/1 -> Controlled Current Source/1
  Voltage Measurement/1 -> Memory/1
  ohms Limiter/1 -> Divide/1
  ohms/1 -> ohms Limiter/1
  connections:
  Lin/RConn1 -- Controlled Current Source/LConn1 -- Voltage Measurement/LConn1 -- Series RLC Branch1/LConn1
  Lout/RConn1 -- Voltage Measurement/LConn2 -- ic(t)/RConn1 -- Series RLC Branch1/RConn1
  Controlled Current Source/RConn1 -- ic(t)/LConn1

== system IEEE_1547_UI_TEST/SM_SystemDynamics/ 3Phase Y Load with N/   R Bank1/R3 ==
  note: I R = V / R
  note: 10
      | Mohms
  ohms : Inport
  Controlled Current Source : powerlib/Electrical Sources/Controlled Current Source  Initialize=on  Source_Type=AC  Amplitude=0  Phase=0  Frequency=0  Measurements=None
      settings: SourceProductName=Simscape Electrical
  Divide : Product  Inputs=/*
  Memory : Memory  InitialCondition=10
  Series RLC Branch1 : powerlib/Elements/Series RLC Branch  LConnTagsString=__new0  RConnTagsString=__new0  BranchType=R  Resistance=10e6  Inductance=1e-3  SetiL0=off  InitialCurrent=0  Capacitance=1e-6  Setx0=off  InitialVoltage=0  Measurements=None
      settings: SourceProductName=Simscape Electrical
  Voltage Measurement : powerlib/Measurements/Voltage Measurement  PhasorSimulation=off  OutputType=Complex  PSBequivalent=0
      settings: SourceProductName=Simscape Electrical
  ic(t) : powerlib/Measurements/Current Measurement  PhasorSimulation=off  OutputType=Complex  PSBequivalent=0
      settings: SourceProductName=Simscape Electrical
  ohms Limiter : Saturate  UpperLimit=100e6  LowerLimit=0.001
  Lin : PMIOPort  Side=Right
  Lout : PMIOPort  Port=2  Side=Right
  V : Outport
  I : Outport  Port=2
  wires:
  Memory/1 -> V/1, Divide/2
  ic(t)/1 -> I/1
  Divide/1 -> Controlled Current Source/1
  Voltage Measurement/1 -> Memory/1
  ohms Limiter/1 -> Divide/1
  ohms/1 -> ohms Limiter/1
  connections:
  Lin/RConn1 -- Controlled Current Source/LConn1 -- Voltage Measurement/LConn1 -- Series RLC Branch1/LConn1
  Lout/RConn1 -- Voltage Measurement/LConn2 -- ic(t)/RConn1 -- Series RLC Branch1/RConn1
  Controlled Current Source/RConn1 -- ic(t)/LConn1

== system IEEE_1547_UI_TEST/SM_SystemDynamics/ 3Phase Y Load with N/( Rint + L ) Bank/AVG( RMS )1 ==
  In1 : Inport
  Mean : powerlib_meascontrol/Measurements/Mean  Freq=60  Vinit=0  Ts=Ts
      settings: SourceProductName=Simscape Electrical
  RMS : powerlib_meascontrol/Measurements/RMS  TrueRMS=on  Freq=60  RMSInit=120  Ts=Ts
      settings: SourceProductName=Simscape Electrical
  Out1 : Outport
  wires:
  Mean/1 -> Out1/1
  RMS/1 -> Mean/1
  In1/1 -> RMS/1

== system IEEE_1547_UI_TEST/SM_SystemDynamics/ 3Phase Y Load with N/( Rint + L ) Bank/L1 ==
  note: di(t)
      | -----
      | dt
  note: L (mH)
  note: v(t)
  note: i(t)
  note: i(t)
  note: Inductor Equations
      |
      | v ( t ) = ( Rint ) i( t ) + L di(t)/dt
      |
      | di(t)/dt = ( 1 / L ) [ v ( t ) - Rint * i ( t ) ]
  note: i(t) * Rint
  mH : Inport
  Rint : Inport  Port=2
  1/L : Product  Inputs=/*  SaturateOnIntegerOverflow=on  OutDataTypeStr=Inherit: Same as first input
  1/L1 : Product  Inputs=**  SaturateOnIntegerOverflow=on  OutDataTypeStr=Inherit: Same as first input
  10 Mohms : powerlib/Elements/Series RLC Branch  LConnTagsString=__new0  RConnTagsString=__new0  BranchType=R  Resistance=10e6  Inductance=1e-3  SetiL0=off  InitialCurrent=0  Capacitance=1e-6  Setx0=off  InitialVoltage=0  Measurements=None
      settings: SourceProductName=Simscape Electrical
  Add : Sum  Inputs=+-
  Constant : Constant  Value=1e-3
  "Inductor current " : powerlib/Electrical Sources/Controlled Current Source  Initialize=on  Source_Type=AC  Amplitude=0  Phase=0  Frequency=0  Measurements=None
      settings: SourceProductName=Simscape Electrical
  Integrator : Integrator
  Vt : powerlib/Measurements/Voltage Measurement  PhasorSimulation=off  OutputType=Magnitude  PSBequivalent=0
      settings: SourceProductName=Simscape Electrical
  i(t) : powerlib/Measurements/Current Measurement  PhasorSimulation=off  OutputType=Complex  PSBequivalent=0
      settings: SourceProductName=Simscape Electrical
  mul1 : Product  Inputs=**  SaturateOnIntegerOverflow=on  OutDataTypeStr=Inherit: Same as first input
  ohms Limiter : Saturate  UpperLimit=inf  LowerLimit=1e-6
  ohms Limiter1 : Saturate  UpperLimit=inf  LowerLimit=1e-6
  + : PMIOPort  Side=Right
  - : PMIOPort  Port=2  Side=Right
  V_L : Outport
  I_L : Outport  Port=2
  wires:
  ohms Limiter1/1 -> mul1/2
  ohms Limiter/1 -> 1/L1/2
  mH/1 -> ohms Limiter/1
  Integrator/1 -> mul1/1, "Inductor current "/1
  Constant/1 -> 1/L1/1
  1/L/1 -> Integrator/1
  mul1/1 -> Add/2
  Rint/1 -> ohms Limiter1/1
  i(t)/1 -> I_L/1
  1/L1/1 -> 1/L/1
  Vt/1 -> V_L/1, Add/1
  Add/1 -> 1/L/2
  connections:
  10 Mohms/RConn1 -- -/RConn1 -- Vt/LConn2 -- "Inductor current "/RConn1
  10 Mohms/LConn1 -- i(t)/LConn1 -- Vt/LConn1 -- +/RConn1
  "Inductor current "/LConn1 -- i(t)/RConn1

== system IEEE_1547_UI_TEST/SM_SystemDynamics/ 3Phase Y Load with N/( Rint + L ) Bank/L2 ==
  note: Inductor Equations
      |
      | v ( t ) = ( Rint ) i( t ) + L di(t)/dt
      |
      | di(t)/dt = ( 1 / L ) [ v ( t ) - Rint * i ( t ) ]
  note: i(t)
  note: i(t) * Rint
  note: v(t)
  note: L (mH)
  note: di(t)
      | -----
      | dt
  note: i(t)
  mH : Inport
  Rint : Inport  Port=2
  1/L : Product  Inputs=/*  SaturateOnIntegerOverflow=on  OutDataTypeStr=Inherit: Same as first input
  1/L1 : Product  Inputs=**  SaturateOnIntegerOverflow=on  OutDataTypeStr=Inherit: Same as first input
  10 Mohms : powerlib/Elements/Series RLC Branch  LConnTagsString=__new0  RConnTagsString=__new0  BranchType=R  Resistance=10e6  Inductance=1e-3  SetiL0=off  InitialCurrent=0  Capacitance=1e-6  Setx0=off  InitialVoltage=0  Measurements=None
      settings: SourceProductName=Simscape Electrical
  Add : Sum  Inputs=+-
  Constant : Constant  Value=1e-3
  "Inductor current " : powerlib/Electrical Sources/Controlled Current Source  Initialize=on  Source_Type=AC  Amplitude=0  Phase=0  Frequency=0  Measurements=None
      settings: SourceProductName=Simscape Electrical
  Integrator : Integrator
  Vt : powerlib/Measurements/Voltage Measurement  PhasorSimulation=off  OutputType=Magnitude  PSBequivalent=0
      settings: SourceProductName=Simscape Electrical
  i(t) : powerlib/Measurements/Current Measurement  PhasorSimulation=off  OutputType=Complex  PSBequivalent=0
      settings: SourceProductName=Simscape Electrical
  mul1 : Product  Inputs=**  SaturateOnIntegerOverflow=on  OutDataTypeStr=Inherit: Same as first input
  ohms Limiter : Saturate  UpperLimit=inf  LowerLimit=1e-6
  ohms Limiter1 : Saturate  UpperLimit=inf  LowerLimit=1e-6
  + : PMIOPort  Side=Right
  - : PMIOPort  Port=2  Side=Right
  V_L : Outport
  I_L : Outport  Port=2
  wires:
  Vt/1 -> V_L/1, Add/1
  Rint/1 -> ohms Limiter1/1
  Add/1 -> 1/L/2
  i(t)/1 -> I_L/1
  Constant/1 -> 1/L1/1
  Integrator/1 -> mul1/1, "Inductor current "/1
  mH/1 -> ohms Limiter/1
  1/L/1 -> Integrator/1
  1/L1/1 -> 1/L/1
  mul1/1 -> Add/2
  ohms Limiter/1 -> 1/L1/2
  ohms Limiter1/1 -> mul1/2
  connections:
  "Inductor current "/RConn1 -- Vt/LConn2 -- -/RConn1 -- 10 Mohms/RConn1
  10 Mohms/LConn1 -- +/RConn1 -- i(t)/LConn1 -- Vt/LConn1
  "Inductor current "/LConn1 -- i(t)/RConn1

== system IEEE_1547_UI_TEST/SM_SystemDynamics/ 3Phase Y Load with N/( Rint + L ) Bank/L3 ==
  note: Inductor Equations
      |
      | v ( t ) = ( Rint ) i( t ) + L di(t)/dt
      |
      | di(t)/dt = ( 1 / L ) [ v ( t ) - Rint * i ( t ) ]
  note: i(t)
  note: i(t) * Rint
  note: v(t)
  note: L (mH)
  note: di(t)
      | -----
      | dt
  note: i(t)
  mH : Inport
  Rint : Inport  Port=2
  1/L : Product  Inputs=/*  SaturateOnIntegerOverflow=on  OutDataTypeStr=Inherit: Same as first input
  1/L1 : Product  Inputs=**  SaturateOnIntegerOverflow=on  OutDataTypeStr=Inherit: Same as first input
  10 Mohms : powerlib/Elements/Series RLC Branch  LConnTagsString=__new0  RConnTagsString=__new0  BranchType=R  Resistance=10e6  Inductance=1e-3  SetiL0=off  InitialCurrent=0  Capacitance=1e-6  Setx0=off  InitialVoltage=0  Measurements=None
      settings: SourceProductName=Simscape Electrical
  Add : Sum  Inputs=+-
  Constant : Constant  Value=1e-3
  "Inductor current " : powerlib/Electrical Sources/Controlled Current Source  Initialize=on  Source_Type=AC  Amplitude=0  Phase=0  Frequency=0  Measurements=None
      settings: SourceProductName=Simscape Electrical
  Integrator : Integrator
  Vt : powerlib/Measurements/Voltage Measurement  PhasorSimulation=off  OutputType=Magnitude  PSBequivalent=0
      settings: SourceProductName=Simscape Electrical
  i(t) : powerlib/Measurements/Current Measurement  PhasorSimulation=off  OutputType=Complex  PSBequivalent=0
      settings: SourceProductName=Simscape Electrical
  mul1 : Product  Inputs=**  SaturateOnIntegerOverflow=on  OutDataTypeStr=Inherit: Same as first input
  ohms Limiter : Saturate  UpperLimit=inf  LowerLimit=1e-6
  ohms Limiter1 : Saturate  UpperLimit=inf  LowerLimit=1e-6
  + : PMIOPort  Side=Right
  - : PMIOPort  Port=2  Side=Right
  V_L : Outport
  I_L : Outport  Port=2
  wires:
  Vt/1 -> V_L/1, Add/1
  Rint/1 -> ohms Limiter1/1
  Add/1 -> 1/L/2
  i(t)/1 -> I_L/1
  Constant/1 -> 1/L1/1
  Integrator/1 -> mul1/1, "Inductor current "/1
  mH/1 -> ohms Limiter/1
  1/L/1 -> Integrator/1
  1/L1/1 -> 1/L/1
  mul1/1 -> Add/2
  ohms Limiter/1 -> 1/L1/2
  ohms Limiter1/1 -> mul1/2
  connections:
  "Inductor current "/RConn1 -- Vt/LConn2 -- -/RConn1 -- 10 Mohms/RConn1
  10 Mohms/LConn1 -- +/RConn1 -- i(t)/LConn1 -- Vt/LConn1
  "Inductor current "/LConn1 -- i(t)/RConn1

== system IEEE_1547_UI_TEST/SM_SystemDynamics/ 3Phase Y Load with N/( Rint + L ) Bank/Power per Element ==
  Vabc : Inport
  Iabc : Inport  Port=2
  Demux : Demux  Outputs=3
  Demux1 : Demux  Outputs=3
  Demux2 : Demux  Outputs=6
  Divide : Product  Inputs=*/
  Gain : Gain  Gain=-1/3
  Mux : Mux  Inputs=6
  Power1 : powerlib_meascontrol/Measurements/Power  Freq=60  Vinit=[1, 0]  Iinit=[1, 0]  Ts=Ts
      settings: SourceProductName=Simscape Power Systems
  Power2 : powerlib_meascontrol/Measurements/Power  Freq=60  Vinit=[1, 0]  Iinit=[1, 0]  Ts=Ts
      settings: SourceProductName=Simscape Power Systems
  Power3 : powerlib_meascontrol/Measurements/Power  Freq=60  Vinit=[1, 0]  Iinit=[1, 0]  Ts=Ts
      settings: SourceProductName=Simscape Power Systems
  tag scope: L1_P=global, L1_Q=global, L2_P=global, L2_Q=global, L3_P=global, L3_Q=global
  wires:
  Demux1/2 -> Power2/2
  Demux/1 -> Power1/1
  Demux1/3 -> Power3/2
  Demux/2 -> Power2/1
  Demux/3 -> Power3/1
  Demux1/1 -> Power1/2
  Iabc/1 -> Demux1/1
  Vabc/1 -> Demux/1
  Demux2/6 -> [L3_Q]
  Power1/1 -> Mux/1
  Power1/2 -> Mux/2
  [Inv_Size] -> Gain/1
  Demux2/3 -> [L2_P]
  Demux2/2 -> [L1_Q]
  Demux2/5 -> [L3_P]
  Demux2/4 -> [L2_Q]
  Divide/1 -> Demux2/1
  Mux/1 -> Divide/1
  Demux2/1 -> [L1_P]
  Power2/1 -> Mux/3
  Power3/2 -> Mux/6
  Power2/2 -> Mux/4
  Power3/1 -> Mux/5
  Gain/1 -> Divide/2

== system IEEE_1547_UI_TEST/SM_SystemDynamics/ 3Phase Y Load with N/( Rint + L ) Bank/Power, 3Ph (  Fund. Frecu. ) ==
  note: Per Unit Converter
  Vabc : Inport
  Iabc : Inport  Port=2
  Divide : Product  Inputs=*/
  Divide1 : Product  Inputs=*/
  Gain : Gain  Gain=-1
  Gain1 : Gain  Gain=-1
  Mean : powerlib_meascontrol/Measurements/Mean  Freq=30  Vinit=0  Ts=Ts
      settings: SourceProductName=Simscape Electrical
  Mean2 : powerlib_meascontrol/Measurements/Mean  Freq=30  Vinit=0  Ts=Ts
      settings: SourceProductName=Simscape Electrical
  PLL (3ph) : powerlib_meascontrol/PLL/PLL (3ph)  Fmin=45  Par_Init=[0, 60]  ParK=[180, 3200, 1]  TcD=1e-4  MaxRateChangeFreq=12  FilterCutOffFreq=25  Ts=Ts  AGC=on
      settings: SourceProductName=Simscape Electrical
  Power ( Fundamental Frecuency ) : powerlib_meascontrol/Measurements/Power (PLL-Driven, Positive-Sequence)  Finit=60  Fmin=60  Vinit=[1, 0]  Iinit=[1, 0]  Ts=Ts
      settings: SourceProductName=Simscape Electrical  SourceProductBaseCode=PS
  P : Outport
  Q : Outport  Port=2
  wires:
  PLL (3ph)/2 -> Power ( Fundamental Frecuency )/2
  PLL (3ph)/1 -> Power ( Fundamental Frecuency )/1
  Iabc/1 -> Power ( Fundamental Frecuency )/4
  Vabc/1 -> PLL (3ph)/1, Power ( Fundamental Frecuency )/3
  Mean/1 -> Divide/1
  [Inv_Size] -> Gain/1
  Gain/1 -> Divide/2
  Power ( Fundamental Frecuency )/2 -> Mean/1
  Divide/1 -> Q/1
  Mean2/1 -> Divide1/1
  [Inv_Size] -> Gain1/1
  Gain1/1 -> Divide1/2
  Power ( Fundamental Frecuency )/1 -> Mean2/1
  Divide1/1 -> P/1

== system IEEE_1547_UI_TEST/SM_SystemDynamics/MASTER CONTROL OUTPUTS/INVERTER MEASURES/Subsystem ==
  trig : Inport
  input : Inport  Port=2
  Constant : Constant  Value=0
  Switch : Switch  Criteria=u2 > Threshold
  Out1 : Outport
  wires:
  Switch/1 -> Out1/1
  trig/1 -> Switch/2
  Constant/1 -> Switch/3
  input/1 -> Switch/1

== system IEEE_1547_UI_TEST/SM_SystemDynamics/MASTER CONTROL OUTPUTS/INVERTER MEASURES/Subsystem1 ==
  trig : Inport
  input : Inport  Port=2
  Constant : Constant  Value=0
  Switch : Switch  Criteria=u2 > Threshold
  Out1 : Outport
  wires:
  Switch/1 -> Out1/1
  trig/1 -> Switch/2
  Constant/1 -> Switch/3
  input/1 -> Switch/1

== system IEEE_1547_UI_TEST/SM_SystemDynamics/OPAL-RT ANALOG INPUTS/Inputs Signal Conditioning Circuit/Subsystem ==
  In : Inport
  "Pha_Comp " : Inport  Port=2
  Add : Sum
  Gain2 : Gain  Gain=pi/180
  PLL (3ph) : powerlib_meascontrol/PLL/PLL (3ph)  Fmin=45  Par_Init=[0, 60]  ParK=[180, 3200, 1]  TcD=1e-4  MaxRateChangeFreq=12  FilterCutOffFreq=25  Ts=Ts  AGC=on
  abc to dq0 : powerlib_meascontrol/Transformations/abc to dq0  Alignment=90 degrees behind phase A axis
  dq0 to abc : powerlib_meascontrol/Transformations/dq0 to abc  Alignment=90 degrees behind phase A axis
  Out : Outport
  wires:
  PLL (3ph)/2 -> abc to dq0/2, Add/1
  "Pha_Comp "/1 -> Gain2/1
  In/1 -> abc to dq0/1, PLL (3ph)/1
  dq0 to abc/1 -> Out/1
  Add/1 -> dq0 to abc/2
  Gain2/1 -> Add/2
  abc to dq0/1 -> dq0 to abc/1

== system IEEE_1547_UI_TEST/SM_SystemDynamics/OPAL-RT ANALOG OUTPUTS/Outputs Signa Conditioning Circuit/Subsystem ==
  trig : Inport
  input : Inport  Port=2
  Constant : Constant  Value=0
  Switch : Switch  Criteria=u2 > Threshold
  Out1 : Outport
  wires:
  Switch/1 -> Out1/1
  trig/1 -> Switch/2
  Constant/1 -> Switch/3
  input/1 -> Switch/1

== system IEEE_1547_UI_TEST/SM_SystemDynamics/OPAL-RT ANALOG OUTPUTS/Outputs Signa Conditioning Circuit/Subsystem1 ==
  trig : Inport
  input : Inport  Port=2
  Constant : Constant  Value=0
  Switch : Switch  Criteria=u2 > Threshold
  Out1 : Outport
  wires:
  Switch/1 -> Out1/1
  trig/1 -> Switch/2
  Constant/1 -> Switch/3
  input/1 -> Switch/1

== system IEEE_1547_UI_TEST/SM_SystemDynamics/OPAL-RT ANALOG OUTPUTS/Outputs Signa Conditioning Circuit/Subsystem2 ==
  trig : Inport
  input : Inport  Port=2
  Constant : Constant  Value=0
  Switch : Switch  Criteria=u2 > Threshold
  Out1 : Outport
  wires:
  Switch/1 -> Out1/1
  trig/1 -> Switch/2
  Constant/1 -> Switch/3
  input/1 -> Switch/1
